simulink model "Maxpid_correction"  (R2015b)
settings: Solver=ode45  StartTime=0.0  StopTime=1  MaxStep=0.01  RelTol=1e-3
undefined symbols (not defined in the file): Cext, Jeq, Kd, Ke, Ki, Kp, R
settings Model: Creator=antomart  LastModifiedBy=David
settings DataIOCC: LimitDataPoints=off  SaveFormat=StructureWithTime
settings HardwareCC: ProdWordSize=32  ProdHWDeviceType=Specified
settings ModelReferenceCC: PropagateSignalLabelsOutOfModel=on
settings GRTTargetCC: GeneratePreprocessorConditionals=Disable all

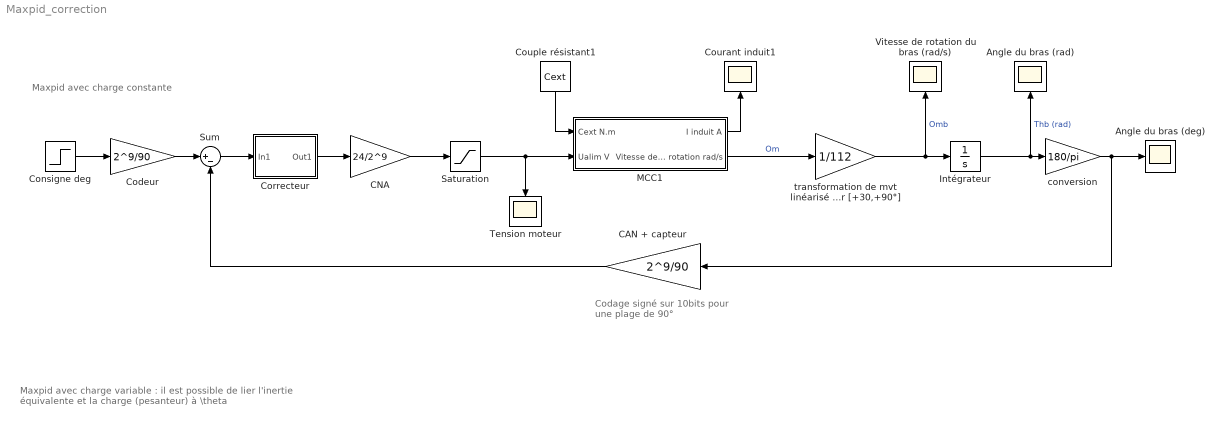
== system Maxpid_correction ==
  note: Maxpid avec charge variable : il est possible de lier l'inertie équivalente et la charge (pesanteur) à \theta
  note: Maxpid avec charge constante
  note: Codage signé sur 10bits pour une plage de 90°
  Angle du bras (rad) : Scope
  Angle du bras (deg) : Scope
  CAN + capteur : Gain  Gain=2^9/90
  CNA : Gain  Gain=24/2^9
  Codeur : Gain  Gain=2^9/90
  Consigne deg : Step  Time=0  After=30  SampleTime=0
  Correcteur : Subsystem
  Couple résistant1 : Constant  Value=Cext
  Courant induit1 : Scope
  Intégrateur : Integrator
  MCC1 : Subsystem
  Saturation : Saturate  UpperLimit=24  LowerLimit=-24
  Sum : Sum  Inputs=|+-
  Tension moteur : Scope
  Vitesse de rotation du bras (rad/s) : Scope
  conversion : Gain  Gain=180/pi
  transformation de mvt linéarisé sur [+30,+90°] : Gain  Gain=1/112
  wires:
  Couple résistant1/1 -> MCC1/1(Cext N.m)
  MCC1/1(I induit A) -> Courant induit1/1
  MCC1/2(Vitesse de rotation rad/s) -> transformation de mvt linéarisé sur [+30,+90°]/1  "Om"
  transformation de mvt linéarisé sur [+30,+90°]/1 -> Intégrateur/1, Vitesse de rotation du bras (rad/s)/1  "Omb"
  Intégrateur/1 -> conversion/1, Angle du bras (rad)/1  "Thb (rad)"
  CNA/1 -> Saturation/1
  Sum/1 -> Correcteur/1(In1)
  Correcteur/1(Out1) -> CNA/1
  Consigne deg/1 -> Codeur/1
  CAN + capteur/1 -> Sum/2
  Codeur/1 -> Sum/1
  conversion/1 -> CAN + capteur/1, Angle du bras (deg)/1
  Saturation/1 -> MCC1/2(Ualim V), Tension moteur/1

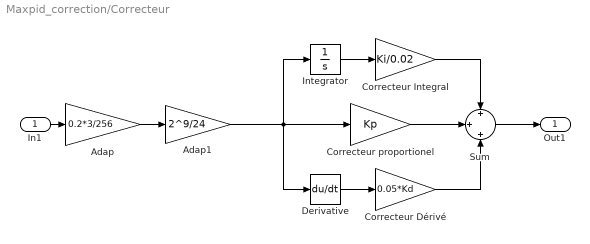
== system Maxpid_correction/Correcteur ==
  In1 : Inport
  Adap : Gain  Gain=0.2*3/256
  Adap1 : Gain  Gain=2^9/24
  Correcteur Dérivé : Gain  Gain=0.05*Kd
  Correcteur Integral : Gain  Gain=Ki/0.02
  Correcteur proportionel : Gain  Gain=Kp
  Derivative : Derivative
  Integrator : Integrator
  Sum : Sum  Inputs=+|+|+
  Out1 : Outport
  wires:
  In1/1 -> Adap/1
  Integrator/1 -> Correcteur Integral/1
  Correcteur Integral/1 -> Sum/1
  Correcteur proportionel/1 -> Sum/2
  Derivative/1 -> Correcteur Dérivé/1
  Correcteur Dérivé/1 -> Sum/3
  Sum/1 -> Out1/1
  Adap/1 -> Adap1/1
  Adap1/1 -> Derivative/1, Integrator/1, Correcteur proportionel/1

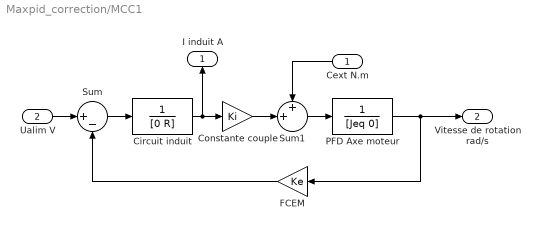
== system Maxpid_correction/MCC1 ==
  Cext N.m : Inport
  Ualim V : Inport  Port=2
  Circuit induit : TransferFcn  Denominator=[0 R]
  Constante couple : Gain  Gain=Ki
  FCEM : Gain  Gain=Ke
  PFD Axe moteur : TransferFcn  Denominator=[Jeq 0]
  Sum : Sum  Inputs=|+-
  Sum1 : Sum  Inputs=++|
  I induit A : Outport
  Vitesse de rotation rad/s : Outport  Port=2
  wires:
  PFD Axe moteur/1 -> Vitesse de rotation rad/s/1, FCEM/1
  Sum1/1 -> PFD Axe moteur/1
  Constante couple/1 -> Sum1/2
  Circuit induit/1 -> Constante couple/1, I induit A/1
  Sum/1 -> Circuit induit/1
  FCEM/1 -> Sum/2
  Cext N.m/1 -> Sum1/1
  Ualim V/1 -> Sum/1
